simulink model "my_io"  (R2025b)
settings: Solver=FixedStepDiscrete  StartTime=0.0  StopTime=10.0  FixedStep=0.02  RelTol=1e-3  EnableMultiTasking=on
libraries: dspnetwork x2, sldrtlib x1
settings Model: Creator=Huawei  LastModifiedBy=lolve
settings OptimizationCC: BlockReduction=off  UseDivisionForNetSlopeComputation=on  OptimizeBlockIOStorage=off

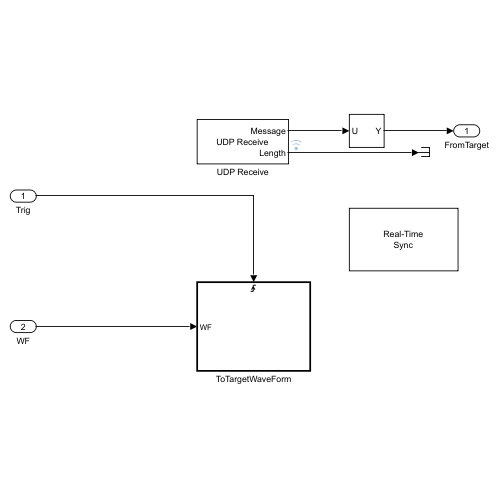
[thumbnail: Simulink's stored preview of the top-level diagram]
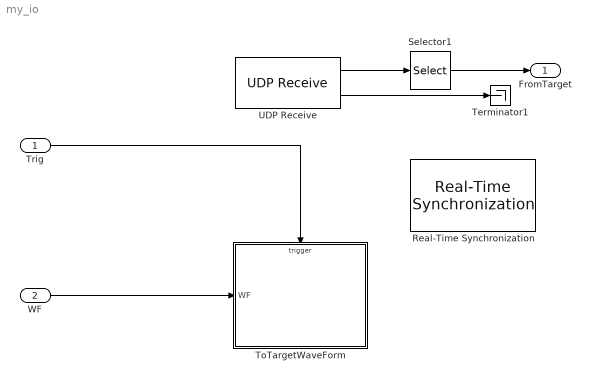
== system my_io ==
  Trig : Inport  OutDataTypeStr=boolean  PortDimensions=1
  WF : Inport  Port=2  OutDataTypeStr=uint16  PortDimensions=20000
  Real-Time Synchronization : sldrtlib/Real-Time Synchronization  SampleTime=0.02  MaxMissedTicks=1000  ShowMissedTicks=off  YieldWhenWaiting=off
  Selector1 : Selector  InputPortWidth=5032  IndexOptions=Index vector (dialog)  Indices=[33:5032]  OutputSizes=1
  Terminator1 : Terminator
  ToTargetWaveForm : Subsystem
  UDP Receive : dspnetwork/UDP Receive  localURL='0.0.0.0'  localPort=25000  remoteURL='0.0.0.0'  remotePort=-1  recvBufferSize=5032*4  dims=5032  signalDatatype=uint16  isComplex=off  isVarSize=off  showBlockingTime=off  blockingTime=0  sampletime=0.02  blockPlatform=[]
      settings: LibrarySourceBlock=dspsrcs4/UDP Receive
  FromTarget : Outport  OutDataTypeStr=uint16  PortDimensions=5000
  wires:
  Trig/1 -> ToTargetWaveForm/Trigger
  WF/1 -> ToTargetWaveForm/1(WF)
  Selector1/1 -> FromTarget/1
  UDP Receive/1 -> Selector1/1
  UDP Receive/2 -> Terminator1/1

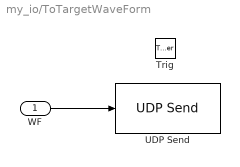
== system my_io/ToTargetWaveForm ==
  WF : Inport  OutDataTypeStr=uint16  PortDimensions=20000
  Trig : TriggerPort  VariantControl=(inherit)  InitialTriggerSignalState=zero  PortDimensions=1
  UDP Send : dspnetwork/UDP Send  remoteURL='127.0.0.1'  remotePort=25002  localURL='0.0.0.0'  localPortSource=Specify via dialog  localPort=25005  sendBufferSize=40000  sampletime=-1  blockPlatform=[]  separateLengthPort=0
      settings: LibrarySourceBlock=dspsnks4/UDP Send
  wires:
  WF/1 -> UDP Send/1
